simulink model "LOPES_3D"  (R2015b)
settings: Solver=ode3  StartTime=0.0  StopTime=inf  FixedStep=ts  RelTol=1e-3
PostLoadFcn:
  | DataFileTemplate = 'd:\%d_LNMC_S01_SLRT_%i.mat';
InitFcn:
  | cd(fileparts(which(gcs)));
  | runScripts
StartFcn:
  | cd(fileparts(which(gcs)));
StopFcn:
  | SaveSLRTData(DataFileTemplate)
values from neighbouring files (symbols this model uses):
  SelectorLOPESInSize = 8    [setAnkleDepInd.m]
libraries: nmc x51, simulink x22, slrtlib x14, LopesDevelopmentLibrary x7, dspsigops x1
(part 2 of 2)

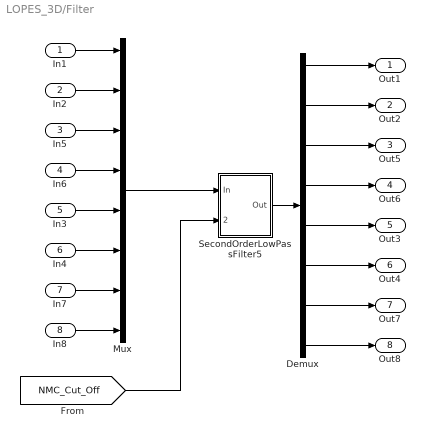
== system LOPES_3D/Filter ==
  In1 : Inport
  In2 : Inport  Port=2
  In5 : Inport  Port=3
  In6 : Inport  Port=4
  In3 : Inport  Port=5
  In4 : Inport  Port=6
  In7 : Inport  Port=7
  In8 : Inport  Port=8
  Demux : Demux  Outputs=8
  Mux : Mux  Inputs=8
  SecondOrderLowPassFilter5 : Subsystem  mask{z=0.7}
      mask prompts: z "Zeta"
  Out1 : Outport
  Out2 : Outport  Port=2
  Out5 : Outport  Port=3
  Out6 : Outport  Port=4
  Out3 : Outport  Port=5
  Out4 : Outport  Port=6
  Out7 : Outport  Port=7
  Out8 : Outport  Port=8
  wires:
  In5/1 -> Mux/3
  In2/1 -> Mux/2
  In1/1 -> Mux/1
  In6/1 -> Mux/4
  In4/1 -> Mux/6
  In3/1 -> Mux/5
  In8/1 -> Mux/8
  In7/1 -> Mux/7
  Mux/1 -> SecondOrderLowPassFilter5/1(In)
  SecondOrderLowPassFilter5/1(Out) -> Demux/1
  Demux/8 -> Out8/1
  Demux/7 -> Out7/1
  Demux/6 -> Out4/1
  Demux/5 -> Out3/1
  Demux/1 -> Out1/1
  Demux/2 -> Out2/1
  Demux/3 -> Out5/1
  Demux/4 -> Out6/1
  [NMC_Cut_Off] -> SecondOrderLowPassFilter5/2(Cut-off (hz))

== system LOPES_3D/FilterEMG ==
  In1 : Inport
  Abs1 : Abs
  SecondOrderHighPassFilter1 : Subsystem  mask{w=10*(2*pi), z=0.7}
      mask prompts: w "Cut off omega [rad/s]"; z "Zeta"
  SecondOrderLowPassFilter2 : LopesDevelopmentLibrary/Various/SecondOrderLowPassFilter  w=10*(2*pi)  z=0.7
  Out1 : Outport
  wires:
  SecondOrderLowPassFilter2/1 -> Out1/1
  Abs1/1 -> SecondOrderLowPassFilter2/1
  SecondOrderHighPassFilter1/1(Out) -> Abs1/1
  In1/1 -> SecondOrderHighPassFilter1/1(In)

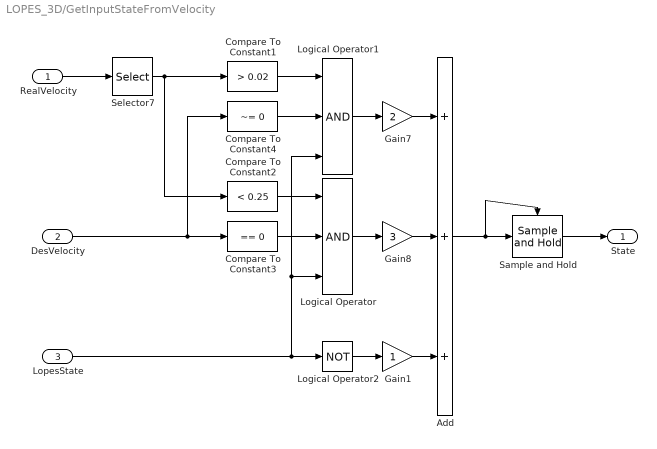
== system LOPES_3D/GetInputStateFromVelocity ==
  RealVelocity : Inport
  DesVelocity : Inport  Port=2
  LopesState : Inport  Port=3
  Add : Sum  Inputs=+++
  Compare To Constant1 : simulink/Logic and Bit Operations/Compare To Constant  relop=>  const=0.02  OutDataTypeStr=boolean
  Compare To Constant2 : simulink/Logic and Bit Operations/Compare To Constant  relop=<  const=0.25  OutDataTypeStr=boolean
  Compare To Constant3 : simulink/Logic and Bit Operations/Compare To Constant  relop===  const=0  OutDataTypeStr=boolean
  Compare To Constant4 : simulink/Logic and Bit Operations/Compare To Constant  relop=~=  const=0  OutDataTypeStr=boolean
  Gain1 : Gain  OutDataTypeStr=double
  Gain7 : Gain  Gain=2  OutDataTypeStr=double
  Gain8 : Gain  Gain=3  OutDataTypeStr=double
  Logical Operator : Logic  Inputs=3  AllPortsSameDT=off  OutDataTypeStr=boolean
  Logical Operator1 : Logic  Inputs=3  AllPortsSameDT=off  OutDataTypeStr=boolean
  Logical Operator2 : Logic  Operator=NOT  AllPortsSameDT=off  OutDataTypeStr=boolean
  Sample and Hold : dspsigops/Sample and Hold  trig=Rising edge  initCond=1  latchinput=off
  Selector7 : Selector  InputPortWidth=7  IndexOptions=Index vector (dialog)  Indices=[2]  OutputSizes=1
  State : Outport
  wires:
  RealVelocity/1 -> Selector7/1
  Selector7/1 -> Compare To Constant2/1, Compare To Constant1/1
  Compare To Constant1/1 -> Logical Operator1/1
  DesVelocity/1 -> Compare To Constant4/1, Compare To Constant3/1
  Compare To Constant3/1 -> Logical Operator/2
  Compare To Constant2/1 -> Logical Operator/1
  Compare To Constant4/1 -> Logical Operator1/2
  Logical Operator1/1 -> Gain7/1
  Logical Operator/1 -> Gain8/1
  Gain7/1 -> Add/1
  Gain8/1 -> Add/2
  Add/1 -> Sample and Hold/Trigger, Sample and Hold/1
  Sample and Hold/1 -> State/1
  LopesState/1 -> Logical Operator1/3, Logical Operator/3, Logical Operator2/1
  Gain1/1 -> Add/3
  Logical Operator2/1 -> Gain1/1

== system LOPES_3D/Label1 ==
  In1 : Inport
  Demux : Demux  Outputs=3
  EstPhase : Concatenate  NumInputs=1
  MeasPhase : Concatenate  NumInputs=1
  Mux : Mux  Inputs=3
  Speed : Concatenate  NumInputs=1
  Out1 : Outport
  wires:
  Mux/1 -> Out1/1
  In1/1 -> Demux/1
  Speed/1 -> Mux/1  "Speed"
  EstPhase/1 -> Mux/3  "EstPhase"
  MeasPhase/1 -> Mux/2  "MeasPhase"
  Demux/1 -> Speed/1
  Demux/2 -> MeasPhase/1
  Demux/3 -> EstPhase/1

== system LOPES_3D/Label4 ==
  In1 : Inport
  Demux : Demux  Outputs=2
  Mux : Mux  Inputs=2
  NMCGain : Concatenate  NumInputs=1
  PosGain : Concatenate  NumInputs=1
  Out1 : Outport
  wires:
  Mux/1 -> Out1/1
  In1/1 -> Demux/1
  PosGain/1 -> Mux/1  "PosGain"
  NMCGain/1 -> Mux/2  "NMCGain"
  Demux/1 -> PosGain/1
  Demux/2 -> NMCGain/1

== system LOPES_3D/Label5 ==
  In1 : Inport
  Angle : Concatenate  NumInputs=1
  Demux : Demux  Outputs=2
  Mux : Mux  Inputs=2
  Phase : Concatenate  NumInputs=1
  Out1 : Outport
  wires:
  Demux/2 -> Phase/1
  Demux/1 -> Angle/1
  Phase/1 -> Mux/2  "Phase"
  Angle/1 -> Mux/1  "Angle"
  In1/1 -> Demux/1
  Mux/1 -> Out1/1

== system LOPES_3D/Label6 ==
  In1 : Inport
  Demux : Demux  Outputs=2
  Force : Concatenate  NumInputs=1
  Mux : Mux  Inputs=2
  Phase : Concatenate  NumInputs=1
  Out1 : Outport
  wires:
  Mux/1 -> Out1/1
  In1/1 -> Demux/1
  Force/1 -> Mux/1  "Force"
  Phase/1 -> Mux/2  "Phase"
  Demux/1 -> Force/1
  Demux/2 -> Phase/1

== system LOPES_3D/LabelAngles ==
  In1 : Inport
  GeyerAngle : Concatenate  NumInputs=1
  Out1 : Outport
  wires:
  In1/1 -> GeyerAngle/1
  GeyerAngle/1 -> Out1/1  "GeyerAngle"

== system LOPES_3D/LabelEMG ==
  Sigs : Inport
  Demux : Demux  Outputs=8
  M{1..8} (8 alike) : Concatenate  NumInputs=1
  Mux1 : Mux  Inputs=8
  LabSigs : Outport
  wires:
  Sigs/1 -> Demux/1
  Demux/1 -> M1/1
  Demux/2 -> M2/1
  Mux1/1 -> LabSigs/1
  Demux/3 -> M3/1
  Demux/4 -> M4/1
  Demux/5 -> M5/1
  Demux/6 -> M6/1
  Demux/7 -> M7/1
  Demux/8 -> M8/1
  M2/1 -> Mux1/2  "M2"
  M1/1 -> Mux1/1  "M1"
  M6/1 -> Mux1/6  "M6"
  M7/1 -> Mux1/7  "M7"
  M3/1 -> Mux1/3  "M3"
  M5/1 -> Mux1/5  "M5"
  M4/1 -> Mux1/4  "M4"
  M8/1 -> Mux1/8  "M8"

== system LOPES_3D/LabelPhase ==
  Sigs : Inport
  Demux : Demux  Outputs=3
  EstPhase : Concatenate  NumInputs=1
  MeasPhase : Concatenate  NumInputs=1
  Mux : Mux  Inputs=3
  Speed : Concatenate  NumInputs=1
  LabSigs : Outport
  wires:
  Demux/3 -> EstPhase/1
  Demux/2 -> MeasPhase/1
  Demux/1 -> Speed/1
  MeasPhase/1 -> Mux/2  "MeasPhase"
  EstPhase/1 -> Mux/3  "EstPhase"
  Speed/1 -> Mux/1  "Speed"
  Sigs/1 -> Demux/1
  Mux/1 -> LabSigs/1

== system LOPES_3D/LabelTorque ==
  In1 : Inport
  NMCTorquePure : Concatenate  NumInputs=1
  Out1 : Outport
  wires:
  NMCTorquePure/1 -> Out1/1  "NMCTorquePure"
  In1/1 -> NMCTorquePure/1

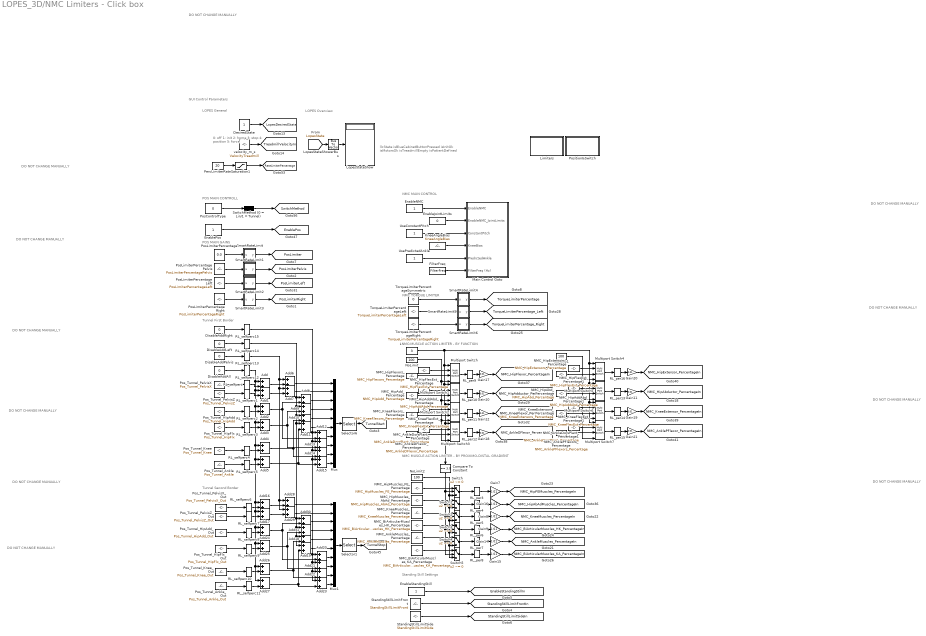
== system LOPES_3D/NMC Limiters - Click box ==
  note: Standing Still Settings
  note: GUI Control Parameters
  note: LOPES Overview
  note: llcState
      | isBlueCabinetButtonPressed
      | isInitOk
      | isMotorsOk
      | isTreadmillEmpty
      | isPatientDefined
  note: 0: off
      | 1: init
      | 2: home
      | 3: stop
      | 4: position
      | 5: force
  note: LOPES General
  note: Tunnel Second Border
  note: POS MAIN CONTROLL
  note: POS MAIN GAINS
  note: NMC MAIN CONTROL
  note: NMC TORQUE LIMITER
  note: NMC MUSCLE ACTION LIMITER - BY PROXIMO-DISTAL GRADIENT
  note: NMC MUSCLE ACTION LIMITER - BY FUNCTION
  note: Tunnel First Border
  note: DO NOT CHANGE MANUALLY
  note: DO NOT CHANGE MANUALLY
  note: DO NOT CHANGE MANUALLY
  note: DO NOT CHANGE MANUALLY
  note: DO NOT CHANGE MANUALLY
  note: DO NOT CHANGE MANUALLY
  note: DO NOT CHANGE MANUALLY
  note: DO NOT CHANGE MANUALLY
  note: DO NOT CHANGE MANUALLY
  note: DO NOT CHANGE MANUALLY
  note: DO NOT CHANGE MANUALLY
  Add{,1..31} (32 alike) : Sum
  Compare To Constant : simulink/Logic and Bit Operations/Compare To Constant  relop===  const=3.0  OutDataTypeStr=boolean
  DesiredState : Constant
  DisableAddAll : Constant  Value=0
  DisableAddLeft : Constant  Value=0
  DisableAddPelvis : Constant  Value=0
  DisableAddRight : Constant  Value=0
  EnableJointLimits : Constant  Value=0  OutDataTypeStr=double
      settings: OpenFcn=|
      | b = get_param(gcb,'value');
      | if (strcmp(b,'1')),
      |   set_param (gcb,'value','0');
      | else
      |   set_param(gcb,'value','1');
      | end;
  EnableNMC : Constant  OutDataTypeStr=double
      settings: OpenFcn=|
      | b = get_param(gcb,'value');
      | if (strcmp(b,'1')),
      |   set_param (gcb,'value','0');
      | else
      |   set_param(gcb,'value','1');
      | end;
  EnablePos : Constant  OutDataTypeStr=double
      settings: OpenFcn=|
      | b = get_param(gcb,'value');
      | if (strcmp(b,'1')),
      |   set_param (gcb,'value','0');
      | else
      |   set_param(gcb,'value','1');
      | end;
  EnableStandingStill : Constant  OutDataTypeStr=double
      settings: OpenFcn=|
      | b = get_param(gcb,'value');
      | if (strcmp(b,'1')),
      |   set_param (gcb,'value','0');
      | else
      |   set_param(gcb,'value','1');
      | end;
  FilterFreq : Constant  Value=FilterFreq
  Gain{7..12,14..21} (14 alike) : Gain  Gain=0.01
  KneeAngleBias : Constant  Value=KneeAngleBias
  LimiterMethod : Constant  Value=3
  Limiters : Subsystem
  LopesStateShow : Display
      settings: AttributesFormatString=%<Tag>
  LopesStateShowerBus : BusToVector
  Main Control Goto : Subsystem
  Multiport Switch{,1..7} (8 alike) : MultiPortSwitch
  Mux : Mux  Inputs=10
  Mux1 : Mux  Inputs=10
  NMC_AnkleDFlexor_Percentage : Constant  Value=NMC_AnkleDFlexor_Percentage
  NMC_AnkleDorsPlant_Percentage : Constant  Value=NMC_AnkleDorsPlant_Percentage
  NMC_AnkleDorsPlant_Percentage1 : Constant  Value=NMC_AnkleDorsPlant_Percentage
  NMC_AnkleMuscles_Percentage : Constant  Value=NMC_AnkleMuscles_Percentage
  NMC_AnklePFlexors_Percentage : Constant  Value=NMC_AnklePFlexors_Percentage
  NMC_BiArticularMuscles_HK_Percentage : Constant  Value=NMC_BiArticularMuscles_HK_Percentage
  NMC_BiArticularMuscles_KA_Percentage : Constant  Value=NMC_BiArticularMuscles_KA_Percentage
  NMC_HipAbd_Percentage : Constant  Value=NMC_HipAbd_Percentage
  NMC_HipAddAbd_Percentage : Constant  Value=NMC_HipAddAbd_Percentage
  NMC_HipAddAbd_Percentage1 : Constant  Value=NMC_HipAddAbd_Percentage
  NMC_HipAdd_Percentage : Constant  Value=NMC_HipAdd_Percentage
  NMC_HipExtensors_Percentage : Constant  Value=NMC_HipExtensors_Percentage
  NMC_HipFlexExt_Percentage : Constant  Value=NMC_HipFlexExt_Percentage
  NMC_HipFlexExt_Percentage1 : Constant  Value=NMC_HipFlexExt_Percentage
  NMC_HipFlexors_Percentage : Constant  Value=NMC_HipFlexors_Percentage
  NMC_HipMuscles_AbAd_Percentage : Constant  Value=NMC_HipMuscles_AbAd_Percentage
  NMC_HipMuscles_FE_Percentage : Constant  Value=NMC_HipMuscles_FE_Percentage
  NMC_KneeExtensors_Percentage : Constant  Value=NMC_KneeExtensors_Percentage
  NMC_KneeFlexExt_Percentage : Constant  Value=NMC_KneeFlexExt_Percentage
  NMC_KneeFlexExt_Percentage1 : Constant  Value=NMC_KneeFlexExt_Percentage
  NMC_KneeFlexors_Percentage : Constant  Value=NMC_KneeFlexors_Percentage
  NMC_KneeMuscles_Percentage : Constant  Value=NMC_KneeMuscles_Percentage
  NoLimit : Constant  Value=100
  NoLimit1 : Constant  Value=100
  NoLimit2 : Constant  Value=100
  PercLimiterRate : Constant  Value=20
  PosControlType : Constant  Value=0  OutDataTypeStr=double
      settings: OpenFcn=|
      | b = get_param(gcb,'value');
      | if (strcmp(b,'1')),
      |   set_param (gcb,'value','0');
      | else
      |   set_param(gcb,'value','1');
      | end;
  PosLimiterPercentage : Constant  Value=0.0
  PosLimiterPercentageLeft : Constant  Value=PosLimiterPercentageLeft
  PosLimiterPercentagePelvis : Constant  Value=PosLimiterPercentagePelvis
  PosLimiterPercentageRight : Constant  Value=PosLimiterPercentageRight
  Pos_Tunnel_Ankle : Constant  Value=Pos_Tunnel_Ankle
  Pos_Tunnel_Ankle_Out : Constant  Value=Pos_Tunnel_Ankle_Out
  Pos_Tunnel_HipAdd : Constant  Value=Pos_Tunnel_HipAdd
  Pos_Tunnel_HipAdd_Out : Constant  Value=Pos_Tunnel_HipAdd_Out
  Pos_Tunnel_HipFlx : Constant  Value=Pos_Tunnel_HipFlx
  Pos_Tunnel_HipFlx_Out : Constant  Value=Pos_Tunnel_HipFlx_Out
  Pos_Tunnel_Knee : Constant  Value=Pos_Tunnel_Knee
  Pos_Tunnel_Knee_Out : Constant  Value=Pos_Tunnel_Knee_Out
  Pos_Tunnel_PelvisX : Constant  Value=Pos_Tunnel_PelvisX
  Pos_Tunnel_PelvisX_Out : Constant  Value=Pos_Tunnel_PelvisX_Out
  Pos_Tunnel_PelvisZ : Constant  Value=Pos_Tunnel_PelvisZ
  Pos_Tunnel_PelvisZ_Out : Constant  Value=Pos_Tunnel_PelvisZ_Out
  Position&Switch : Subsystem
  RL_per{3..16} (14 alike) : nmc/RL_per
  RL_selfperc{,1..15} (16 alike) : nmc/RL_selfperc
  Saturation1 : Saturate  UpperLimit=100  LowerLimit=0
  Selector1 : Selector  InputPortWidth=10  IndexOptions=Index vector (dialog)  Indices=SelectorLOPESIn  OutputSizes=1
  Selector6 : Selector  InputPortWidth=10  IndexOptions=Index vector (dialog)  Indices=SelectorLOPESIn  OutputSizes=1
  SmartRateLimit : Subsystem
  SmartRateLimit1 : Subsystem
  SmartRateLimit2 : Subsystem
  SmartRateLimit3 : Subsystem
  SmartRateLimit4 : Subsystem
  SmartRateLimit5 : Subsystem
  SmartRateLimit6 : Subsystem
  StandingStillLimitFront : Constant  Value=StandingStillLimitFront
  StandingStillLimitSide : Constant  Value=StandingStillLimitSide
  Switch{,1..5} (6 alike) : Switch  Criteria=u2 ~= 0
  SwitchMethod (0 = Lin/1 = Tunnel) : Concatenate  NumInputs=1
  TorqueLimiterPercentageLeft : Constant  Value=TorqueLimiterPercentageLeft
  TorqueLimiterPercentageRight : Constant  Value=TorqueLimiterPercentageRight
  TorqueLimiterPercentageSymmetric : Constant  Value=0
  UseConstantPitch : Constant  OutDataTypeStr=double
      settings: OpenFcn=|
      | b = get_param(gcb,'value');
      | if (strcmp(b,'1')),
      |   set_param (gcb,'value','0');
      | else
      |   set_param(gcb,'value','1');
      | end;
  UsePredictedAnkle : Constant  OutDataTypeStr=double
      settings: OpenFcn=|
      | b = get_param(gcb,'value');
      | if (strcmp(b,'1')),
      |   set_param (gcb,'value','0');
      | else
      |   set_param(gcb,'value','1');
      | end;
  velocity_m_s : Constant  Value=VelocityTreadmill
  tag scope: EnablePos=global, EnableStandingStillIn=global, LopesDesiredState=global, NMC_AnkleDFlexor_PercentageIn=global, NMC_AnkleMuscles_PercentageIn=global, NMC_AnklePFlexor_PercentageIn=global, NMC_BiArticularMuscles_HK_PercentageIn=global, NMC_BiArticularMuscles_KA_PercentageIn=global, NMC_HipAbAdMuscles_PercentageIn=global, NMC_HipAbductor_PercentageIn=global, NMC_HipAdductor_PercentageIn=global, NMC_HipExtensor_PercentageIn=global, NMC_HipFEMuscles_PercentageIn=global, NMC_HipFlexor_PercentageIn=global, NMC_KneeExtensor_PercentageIn=global, NMC_KneeFlexor_PercentageIn=global, NMC_KneeMuscles_PercentageIn=global, PosLimiter=global, PosLimiterLeft=global, PosLimiterPelvis=global, PosLimiterRight=global, RateLimiterPercentage=global, StandingStillLimitFrontIn=global, StandingStillLimitSideIn=global, SwitchMethod=global, TorqueLimiterPercentage=global, TorqueLimiterPercentage_Left=global, TorqueLimiterPercentage_Right=global, TreadmillVelocityIn=global, TunnelStart=global, TunnelStop=global
  wires:
  Switch5/1 -> RL_per8/1
  Switch4/1 -> RL_per7/1
  Switch3/1 -> RL_per6/1
  Switch/1 -> RL_per3/1
  Switch1/1 -> RL_per4/1
  Switch2/1 -> RL_per5/1
  NMC_BiArticularMuscles_KA_Percentage/1 -> Switch5/1
  NMC_AnkleMuscles_Percentage/1 -> Switch4/1
  NMC_BiArticularMuscles_HK_Percentage/1 -> Switch3/1
  NMC_KneeMuscles_Percentage/1 -> Switch2/1
  NMC_HipMuscles_AbAd_Percentage/1 -> Switch1/1
  NoLimit2/1 -> Switch/3, Switch1/3, Switch2/3, Switch3/3, Switch4/3, Switch5/3
  NoLimit/1 -> Multiport Switch2/4, Multiport Switch3/4, Multiport Switch1/4, Multiport Switch/4
  NMC_HipFlexExt_Percentage1/1 -> Multiport Switch4/2
  NMC_HipAddAbd_Percentage1/1 -> Multiport Switch5/2
  NMC_KneeFlexExt_Percentage1/1 -> Multiport Switch6/2
  NMC_AnkleDorsPlant_Percentage1/1 -> Multiport Switch7/2
  NMC_HipFlexExt_Percentage/1 -> Multiport Switch/2
  NMC_KneeFlexExt_Percentage/1 -> Multiport Switch2/2
  NMC_AnkleDorsPlant_Percentage/1 -> Multiport Switch3/2
  NMC_HipAddAbd_Percentage/1 -> Multiport Switch1/2
  NoLimit1/1 -> Multiport Switch7/4, Multiport Switch6/4, Multiport Switch5/4, Multiport Switch4/4
  Multiport Switch7/1 -> RL_per15/1
  Multiport Switch6/1 -> RL_per14/1
  Multiport Switch5/1 -> RL_per13/1
  Multiport Switch4/1 -> RL_per16/1
  NMC_AnklePFlexors_Percentage/1 -> Multiport Switch7/3
  NMC_KneeExtensors_Percentage/1 -> Multiport Switch6/3
  NMC_HipAbd_Percentage/1 -> Multiport Switch5/3
  NMC_HipExtensors_Percentage/1 -> Multiport Switch4/3
  NMC_AnkleDFlexor_Percentage/1 -> Multiport Switch3/3
  Multiport Switch3/1 -> RL_per12/1
  Multiport Switch2/1 -> RL_per11/1
  Multiport Switch1/1 -> RL_per10/1
  Multiport Switch/1 -> RL_per9/1
  LimiterMethod/1 -> Multiport Switch4/1, Multiport Switch5/1, Multiport Switch6/1, Multiport Switch7/1, Multiport Switch2/1, Compare To Constant/1, Multiport Switch3/1, Multiport Switch1/1, Multiport Switch/1
  SmartRateLimit4/1(y) -> [TorqueLimiterPercentage]
  TorqueLimiterPercentageSymmetric/1 -> SmartRateLimit4/1(u)
  SmartRateLimit/1(y) -> [PosLimiter]
  PosLimiterPercentage/1 -> SmartRateLimit/1(u)
  StandingStillLimitFront/1 -> [StandingStillLimitFrontIn]
  StandingStillLimitSide/1 -> [StandingStillLimitSideIn]
  EnableStandingStill/1 -> [EnableStandingStillIn]
  [LopesState] -> LopesStateShowerBus/1
  LopesStateShowerBus/1 -> LopesStateShow/1
  DesiredState/1 -> [LopesDesiredState]
  velocity_m_s/1 -> [TreadmillVelocityIn]
  Mux1/1 -> Selector1/1
  Pos_Tunnel_PelvisX_Out/1 -> RL_selfperc6/1
  Pos_Tunnel_Ankle_Out/1 -> RL_selfperc11/1
  Pos_Tunnel_Knee_Out/1 -> RL_selfperc10/1
  Pos_Tunnel_HipFlx_Out/1 -> RL_selfperc9/1
  Pos_Tunnel_HipAdd_Out/1 -> RL_selfperc8/1
  Pos_Tunnel_PelvisZ_Out/1 -> RL_selfperc7/1
  RL_selfperc/1 -> Add/2
  RL_selfperc1/1 -> Add1/2
  Mux/1 -> Selector6/1
  Pos_Tunnel_PelvisX/1 -> RL_selfperc/1
  Selector6/1 -> [TunnelStart]
  Pos_Tunnel_Ankle/1 -> RL_selfperc5/1
  Pos_Tunnel_Knee/1 -> RL_selfperc4/1
  Pos_Tunnel_HipFlx/1 -> RL_selfperc3/1
  Pos_Tunnel_HipAdd/1 -> RL_selfperc2/1
  Pos_Tunnel_PelvisZ/1 -> RL_selfperc1/1
  EnablePos/1 -> [EnablePos]
  SwitchMethod (0 = Lin/1 = Tunnel)/1 -> [SwitchMethod]
  Saturation1/1 -> [RateLimiterPercentage]
  PercLimiterRate/1 -> Saturation1/1
  Selector1/1 -> [TunnelStop]
  PosControlType/1 -> SwitchMethod (0 = Lin/1 = Tunnel)/1
  SmartRateLimit1/1(y) -> [PosLimiterPelvis]
  PosLimiterPercentagePelvis/1 -> SmartRateLimit1/1(u)
  PosLimiterPercentageRight/1 -> SmartRateLimit3/1(u)
  SmartRateLimit3/1(y) -> [PosLimiterRight]
  SmartRateLimit2/1(y) -> [PosLimiterLeft]
  PosLimiterPercentageLeft/1 -> SmartRateLimit2/1(u)
  FilterFreq/1 -> Main Control Goto/6(FilterFreq (Hz))
  UsePredictedAnkle/1 -> Main Control Goto/5(PredictedAnkle)
  KneeAngleBias/1 -> Main Control Goto/4("KneeBias ")
  UseConstantPitch/1 -> Main Control Goto/3(ConstantPitch)
  EnableJointLimits/1 -> Main Control Goto/2(EnableNMC_JointLimits)
  EnableNMC/1 -> Main Control Goto/1(EnableNMC)
  TorqueLimiterPercentageRight/1 -> SmartRateLimit6/1(u)
  TorqueLimiterPercentageLeft/1 -> SmartRateLimit5/1(u)
  RL_per8/1 -> Gain15/1
  RL_per7/1 -> Gain14/1
  RL_per6/1 -> Gain9/1
  RL_per5/1 -> Gain8/1
  RL_per4/1 -> Gain16/1
  RL_per3/1 -> Gain7/1
  Gain16/1 -> [NMC_HipAbAdMuscles_PercentageIn]
  Gain15/1 -> [NMC_BiArticularMuscles_KA_PercentageIn]
  Gain14/1 -> [NMC_AnkleMuscles_PercentageIn]
  Gain9/1 -> [NMC_BiArticularMuscles_HK_PercentageIn]
  Gain8/1 -> [NMC_KneeMuscles_PercentageIn]
  Gain7/1 -> [NMC_HipFEMuscles_PercentageIn]
  NMC_HipMuscles_FE_Percentage/1 -> Switch/1
  RL_per15/1 -> Gain21/1
  RL_per14/1 -> Gain19/1
  RL_per16/1 -> Gain20/1
  RL_per13/1 -> Gain11/1
  RL_per12/1 -> Gain18/1
  RL_per11/1 -> Gain12/1
  NMC_KneeFlexors_Percentage/1 -> Multiport Switch2/3
  RL_per10/1 -> Gain10/1
  NMC_HipAdd_Percentage/1 -> Multiport Switch1/3
  RL_per9/1 -> Gain17/1
  NMC_HipFlexors_Percentage/1 -> Multiport Switch/3
  Gain11/1 -> [NMC_HipAbductor_PercentageIn]
  Gain10/1 -> [NMC_HipAdductor_PercentageIn]
  Gain21/1 -> [NMC_AnklePFlexor_PercentageIn]
  Gain20/1 -> [NMC_HipExtensor_PercentageIn]
  Gain19/1 -> [NMC_KneeExtensor_PercentageIn]
  Gain18/1 -> [NMC_AnkleDFlexor_PercentageIn]
  Gain17/1 -> [NMC_HipFlexor_PercentageIn]
  Gain12/1 -> [NMC_KneeFlexor_PercentageIn]
  Compare To Constant/1 -> Switch5/2, Switch4/2, Switch3/2, Switch2/2, Switch1/2, Switch/2
  DisableAddAll/1 -> RL_selfperc12/1
  DisableAddPelvis/1 -> RL_selfperc13/1
  DisableAddLeft/1 -> RL_selfperc14/1
  DisableAddRight/1 -> RL_selfperc15/1
  Add/1 -> Add6/2
  RL_selfperc2/1 -> Add2/2
  Add2/1 -> Add12/2, Add8/2
  RL_selfperc3/1 -> Add3/2
  Add3/1 -> Add9/2, Add13/2
  RL_selfperc4/1 -> Add4/2
  Add4/1 -> Add14/2, Add10/2
  RL_selfperc5/1 -> Add5/2
  Add5/1 -> Add15/2, Add11/2
  Add6/1 -> Mux/1
  Add1/1 -> Add7/2
  Add7/1 -> Mux/2
  Add8/1 -> Mux/3
  Add9/1 -> Mux/4
  Add10/1 -> Mux/5
  Add11/1 -> Mux/6
  Add12/1 -> Mux/7
  Add13/1 -> Mux/8
  Add14/1 -> Mux/9
  Add15/1 -> Mux/10
  RL_selfperc6/1 -> Add16/2
  RL_selfperc7/1 -> Add17/2
  Add16/1 -> Add28/2
  RL_selfperc12/1 -> Add1/1, Add16/1, Add24/1, Add25/1, Add26/1, Add27/1, Add17/1, Add5/1, Add4/1, Add3/1, Add2/1, Add/1
  RL_selfperc8/1 -> Add24/2
  Add24/1 -> Add30/2, Add20/2
  RL_selfperc9/1 -> Add25/2
  Add25/1 -> Add21/2, Add31/2
  RL_selfperc10/1 -> Add26/2
  Add26/1 -> Add18/2, Add22/2
  RL_selfperc11/1 -> Add27/2
  Add27/1 -> Add19/2, Add23/2
  RL_selfperc13/1 -> Add28/1, Add29/1, Add7/1, Add6/1
  Add28/1 -> Mux1/1
  Add17/1 -> Add29/2
  Add29/1 -> Mux1/2
  RL_selfperc14/1 -> Add30/1, Add31/1, Add18/1, Add19/1, Add11/1, Add10/1, Add9/1, Add8/1
  Add30/1 -> Mux1/3
  Add31/1 -> Mux1/4
  Add18/1 -> Mux1/5
  Add19/1 -> Mux1/6
  Add20/1 -> Mux1/7
  Add21/1 -> Mux1/8
  Add22/1 -> Mux1/9
  Add23/1 -> Mux1/10
  RL_selfperc15/1 -> Add20/1, Add21/1, Add22/1, Add23/1, Add15/1, Add14/1, Add13/1, Add12/1
  SmartRateLimit5/1(y) -> [TorqueLimiterPercentage_Left]
  SmartRateLimit6/1(y) -> [TorqueLimiterPercentage_Right]

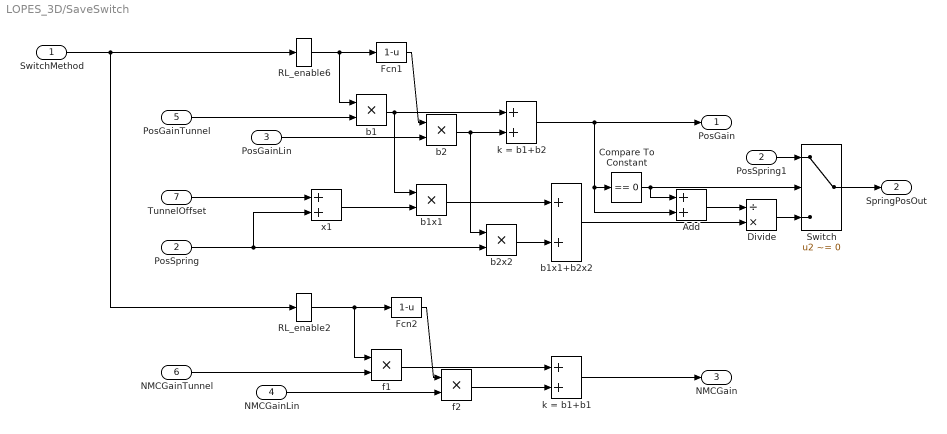
== system LOPES_3D/SaveSwitch ==
  SwitchMethod : Inport
  PosSpring : Inport  Port=2
  PosGainLin : Inport  Port=3
  NMCGainLin : Inport  Port=4
  PosGainTunnel : Inport  Port=5
  NMCGainTunnel : Inport  Port=6
  "TunnelOffset " : Inport  Port=7
  Add : Sum
  Compare To Constant : simulink/Logic and Bit Operations/Compare To Constant  relop===  const=0  OutDataTypeStr=boolean
  Divide : Product  Inputs=/*
  Fcn1 : Fcn  Expr=1-u
  Fcn2 : Fcn  Expr=1-u
  PosSpring1 : InportShadow  Port=2
  RL_enable2 : nmc/RL_enable
  RL_enable6 : nmc/RL_enable
  Switch : Switch  Criteria=u2 ~= 0
  b1 : Product
  b1x1 : Product
  b1x1+b2x2 : Sum
  b2 : Product
  b2x2 : Product
  f1 : Product
  f2 : Product
  k = b1+b1 : Sum
  k = b1+b2 : Sum
  x1 : Sum
  PosGain : Outport
  SpringPosOut : Outport  Port=2
  NMCGain : Outport  Port=3
  wires:
  RL_enable6/1 -> b1/1, Fcn1/1
  k = b1+b2/1 -> PosGain/1, Add/2, Compare To Constant/1
  NMCGainTunnel/1 -> f1/2
  b1x1+b2x2/1 -> Divide/2
  f1/1 -> k = b1+b1/1
  b2x2/1 -> b1x1+b2x2/2
  "TunnelOffset "/1 -> x1/1
  PosSpring/1 -> x1/2, b2x2/2
  x1/1 -> b1x1/2
  SwitchMethod/1 -> RL_enable2/1, RL_enable6/1
  Fcn2/1 -> f2/1
  RL_enable2/1 -> Fcn2/1, f1/1
  NMCGainLin/1 -> f2/2
  b2/1 -> b2x2/1, k = b1+b2/2
  b1x1/1 -> b1x1+b2x2/1
  b1/1 -> b1x1/1, k = b1+b2/1
  k = b1+b1/1 -> NMCGain/1
  f2/1 -> k = b1+b1/2
  PosGainTunnel/1 -> b1/2
  Fcn1/1 -> b2/1
  PosGainLin/1 -> b2/2
  Compare To Constant/1 -> Switch/2, Add/1
  Switch/1 -> SpringPosOut/1
  PosSpring1/1 -> Switch/1
  Divide/1 -> Switch/3
  Add/1 -> Divide/1

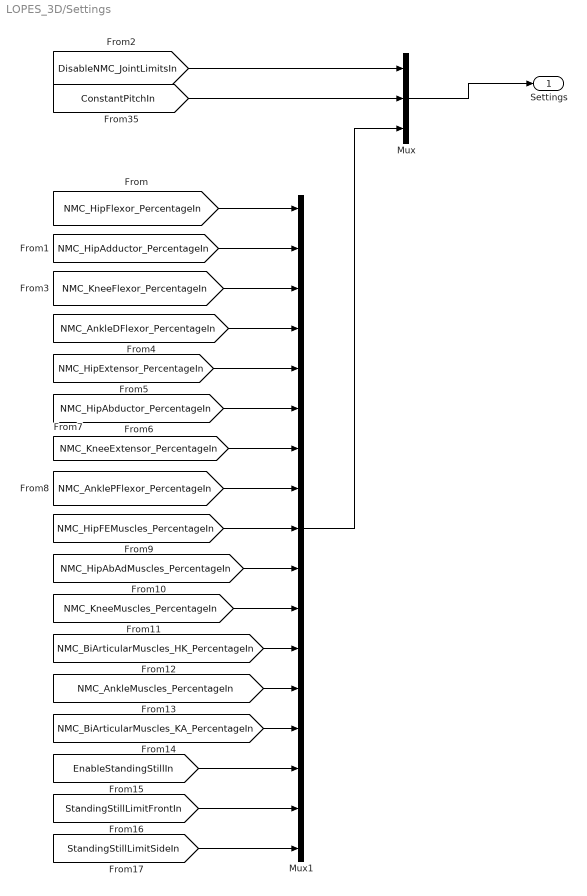
== system LOPES_3D/Settings ==
  Mux : Mux  Inputs=3
  Mux1 : Mux  Inputs=17
  Settings : Outport
  wires:
  [ConstantPitchIn] -> Mux/2
  [DisableNMC_JointLimitsIn] -> Mux/1
  Mux/1 -> Settings/1
  [NMC_BiArticularMuscles_HK_PercentageIn] -> Mux1/12
  [NMC_BiArticularMuscles_KA_PercentageIn] -> Mux1/14
  [NMC_AnkleMuscles_PercentageIn] -> Mux1/13
  [NMC_HipAbAdMuscles_PercentageIn] -> Mux1/10
  [NMC_HipAdductor_PercentageIn] -> Mux1/2
  [NMC_HipFEMuscles_PercentageIn] -> Mux1/9
  [NMC_AnklePFlexor_PercentageIn] -> Mux1/8
  [NMC_KneeFlexor_PercentageIn] -> Mux1/3
  [NMC_AnkleDFlexor_PercentageIn] -> Mux1/4
  [NMC_HipAbductor_PercentageIn] -> Mux1/6
  [NMC_KneeMuscles_PercentageIn] -> Mux1/11
  [NMC_HipExtensor_PercentageIn] -> Mux1/5
  [NMC_KneeExtensor_PercentageIn] -> Mux1/7
  [NMC_HipFlexor_PercentageIn] -> Mux1/1
  Mux1/1 -> Mux/3
  [EnableStandingStillIn] -> Mux1/15
  [StandingStillLimitFrontIn] -> Mux1/16
  [StandingStillLimitSideIn] -> Mux1/17

== system LOPES_3D/Simple Linear Switch ==
  ones : Constant  Value=ones(SelectorLOPESInSize,1)
  pos_gain : Outport
  NMC_gain : Outport  Port=2
  wires:
  ones/1 -> NMC_gain/1, pos_gain/1

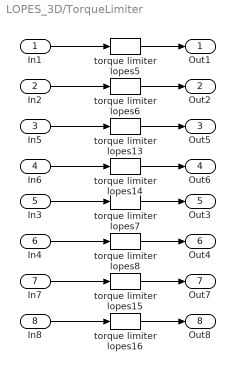
== system LOPES_3D/TorqueLimiter ==
  In1 : Inport
  In2 : Inport  Port=2
  In5 : Inport  Port=3
  In6 : Inport  Port=4
  In3 : Inport  Port=5
  In4 : Inport  Port=6
  In7 : Inport  Port=7
  In8 : Inport  Port=8
  torque limiter lopes{5..6,13..14} (4 alike) : nmc/torque limiter lopes  TorqueLimiterPercentage=TorqueLimiterPercentage_Right
  torque limiter lopes{7..8,15..16} (4 alike) : nmc/torque limiter lopes  TorqueLimiterPercentage=TorqueLimiterPercentage_Left
  Out1 : Outport
  Out2 : Outport  Port=2
  Out5 : Outport  Port=3
  Out6 : Outport  Port=4
  Out3 : Outport  Port=5
  Out4 : Outport  Port=6
  Out7 : Outport  Port=7
  Out8 : Outport  Port=8
  wires:
  In1/1 -> torque limiter lopes5/1
  In3/1 -> torque limiter lopes7/1
  In2/1 -> torque limiter lopes6/1
  In4/1 -> torque limiter lopes8/1
  torque limiter lopes5/1 -> Out1/1
  torque limiter lopes6/1 -> Out2/1
  torque limiter lopes7/1 -> Out3/1
  torque limiter lopes8/1 -> Out4/1
  In5/1 -> torque limiter lopes13/1
  In7/1 -> torque limiter lopes15/1
  In6/1 -> torque limiter lopes14/1
  In8/1 -> torque limiter lopes16/1
  torque limiter lopes13/1 -> Out5/1
  torque limiter lopes14/1 -> Out6/1
  torque limiter lopes15/1 -> Out7/1
  torque limiter lopes16/1 -> Out8/1

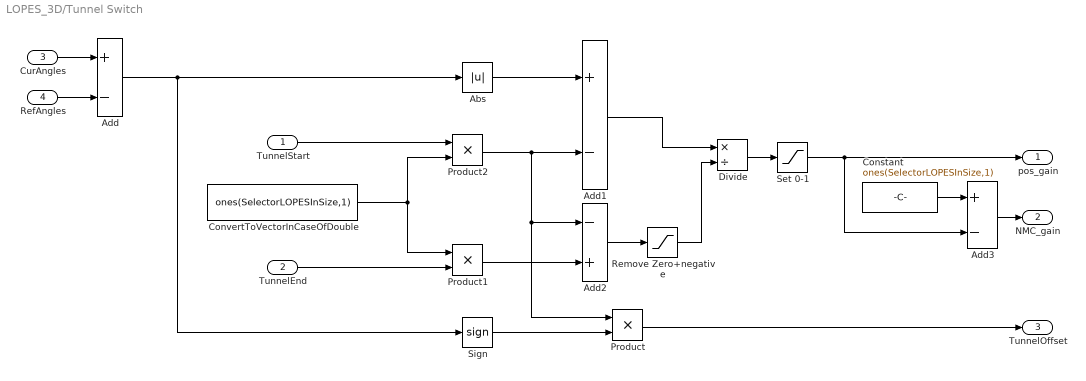
== system LOPES_3D/Tunnel Switch ==
  TunnelStart : Inport
  TunnelEnd : Inport  Port=2
  CurAngles : Inport  Port=3
  RefAngles : Inport  Port=4
  Abs : Abs
  Add : Sum  Inputs=+-
  Add1 : Sum  Inputs=+-
  Add2 : Sum  Inputs=-+
  Add3 : Sum  Inputs=+-
  Constant : Constant  Value=ones(SelectorLOPESInSize,1)
  ConvertToVectorInCaseOfDouble : Constant  Value=ones(SelectorLOPESInSize,1)
  Divide : Product  Inputs=*/
  Product : Product
  Product1 : Product
  Product2 : Product
  Remove Zero+negative : Saturate  UpperLimit=inf  LowerLimit=0.00001  LinearizeAsGain=off
  "Set 0-1 " : Saturate  UpperLimit=1  LowerLimit=0  LinearizeAsGain=off
  Sign : Signum
  pos_gain : Outport
  NMC_gain : Outport  Port=2
  TunnelOffset : Outport  Port=3
  wires:
  CurAngles/1 -> Add/1
  RefAngles/1 -> Add/2
  Add/1 -> Abs/1, Sign/1
  Abs/1 -> Add1/1
  Add1/1 -> Divide/1
  Divide/1 -> "Set 0-1 "/1
  "Set 0-1 "/1 -> pos_gain/1, Add3/2
  Add2/1 -> Remove Zero+negative/1
  Remove Zero+negative/1 -> Divide/2
  Constant/1 -> Add3/1
  Add3/1 -> NMC_gain/1
  Sign/1 -> Product/2
  Product/1 -> TunnelOffset/1
  TunnelEnd/1 -> Product1/2
  ConvertToVectorInCaseOfDouble/1 -> Product1/1, Product2/2
  Product1/1 -> Add2/2
  TunnelStart/1 -> Product2/1
  Product2/1 -> Product/1, Add2/1, Add1/2

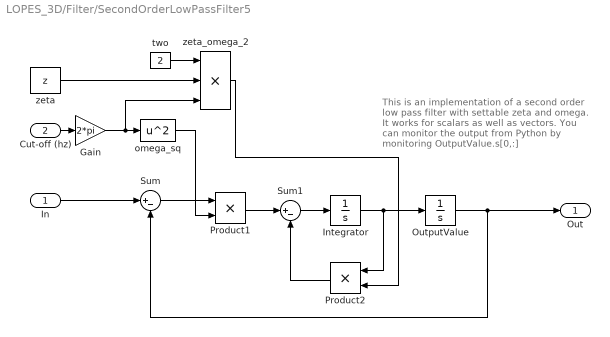
== system LOPES_3D/Filter/SecondOrderLowPassFilter5 ==
  note: This is an implementation of a
      | second order low pass filter with
      | settable zeta and omega.
      | It works for scalars as well as vectors.
      |
      | You can monitor the output from Python
      | by monitoring OutputValue.s[0,:]
  In : Inport
  Cut-off (hz) : Inport  Port=2
  Gain : Gain  Gain=2*pi
  Integrator : Integrator
  OutputValue : Integrator
  Product1 : Product  RndMeth=Zero
  Product2 : Product  RndMeth=Zero
  Sum : Sum  Inputs=|+-
  Sum1 : Sum  Inputs=|+-
  omega_sq : Math  Operator=square  SaturateOnIntegerOverflow=on
  two : Constant  Value=2
  zeta : Constant  Value=z
  zeta_omega_2 : Product  Inputs=3  RndMeth=Zero
  Out : Outport
  wires:
  Product2/1 -> Sum1/2
  zeta_omega_2/1 -> Product2/2
  Product1/1 -> Sum1/1
  omega_sq/1 -> Product1/2
  zeta/1 -> zeta_omega_2/2
  two/1 -> zeta_omega_2/1
  Cut-off (hz)/1 -> Gain/1
  Sum/1 -> Product1/1
  Integrator/1 -> OutputValue/1, Product2/1
  In/1 -> Sum/1
  Sum1/1 -> Integrator/1
  OutputValue/1 -> Sum/2, Out/1
  Gain/1 -> omega_sq/1, zeta_omega_2/3

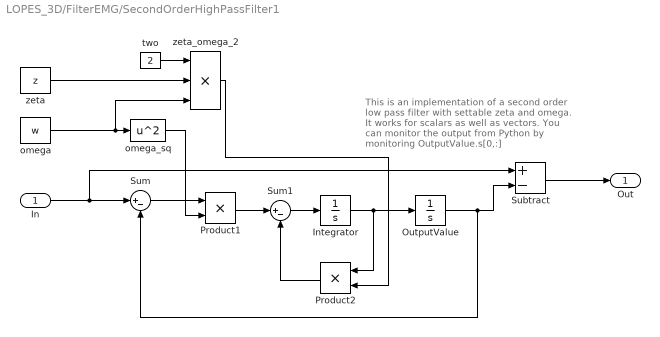
== system LOPES_3D/FilterEMG/SecondOrderHighPassFilter1 ==
  note: This is an implementation of a
      | second order low pass filter with
      | settable zeta and omega.
      | It works for scalars as well as vectors.
      |
      | You can monitor the output from Python
      | by monitoring OutputValue.s[0,:]
  In : Inport
  Integrator : Integrator
  OutputValue : Integrator
  Product1 : Product  RndMeth=Zero
  Product2 : Product  RndMeth=Zero
  Subtract : Sum  Inputs=+-
  Sum : Sum  Inputs=|+-
  Sum1 : Sum  Inputs=|+-
  omega : Constant  Value=w
  omega_sq : Math  Operator=square  SaturateOnIntegerOverflow=on
  two : Constant  Value=2
  zeta : Constant  Value=z
  zeta_omega_2 : Product  Inputs=3  RndMeth=Zero
  Out : Outport
  wires:
  Product2/1 -> Sum1/2
  zeta_omega_2/1 -> Product2/2
  Product1/1 -> Sum1/1
  omega_sq/1 -> Product1/2
  zeta/1 -> zeta_omega_2/2
  two/1 -> zeta_omega_2/1
  omega/1 -> omega_sq/1, zeta_omega_2/3
  Sum/1 -> Product1/1
  Integrator/1 -> OutputValue/1, Product2/1
  In/1 -> Subtract/1, Sum/1
  Sum1/1 -> Integrator/1
  OutputValue/1 -> Subtract/2, Sum/2
  Subtract/1 -> Out/1

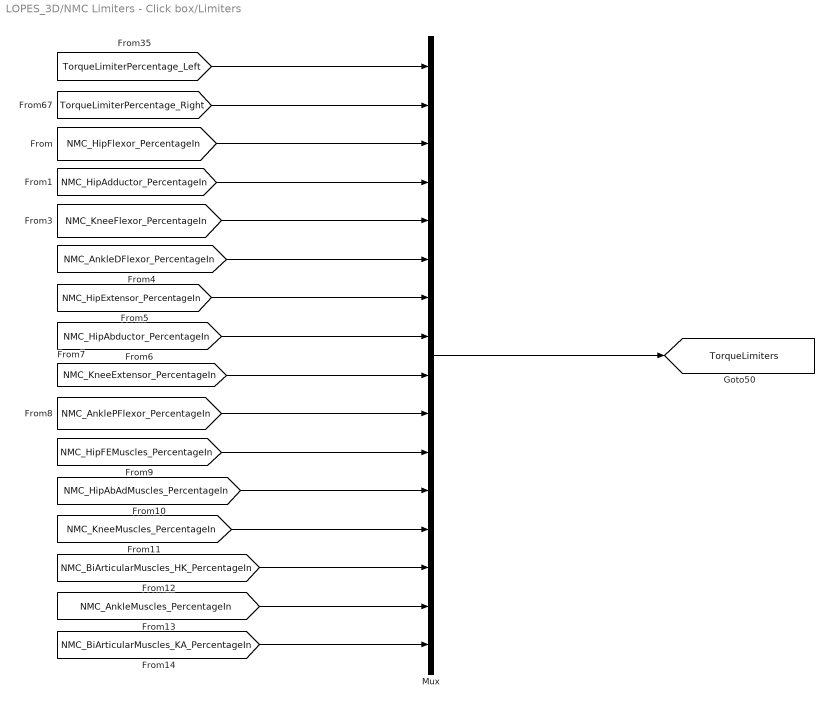
== system LOPES_3D/NMC Limiters - Click box/Limiters ==
  Mux : Mux  Inputs=16
  tag scope: TorqueLimiters=global
  wires:
  [NMC_HipExtensor_PercentageIn] -> Mux/7
  [TorqueLimiterPercentage_Left] -> Mux/1
  [NMC_HipAdductor_PercentageIn] -> Mux/4
  [NMC_HipFlexor_PercentageIn] -> Mux/3
  [TorqueLimiterPercentage_Right] -> Mux/2
  [NMC_AnklePFlexor_PercentageIn] -> Mux/10
  [NMC_KneeFlexor_PercentageIn] -> Mux/5
  [NMC_HipFEMuscles_PercentageIn] -> Mux/11
  [NMC_HipAbductor_PercentageIn] -> Mux/8
  [NMC_AnkleDFlexor_PercentageIn] -> Mux/6
  [NMC_KneeExtensor_PercentageIn] -> Mux/9
  [NMC_KneeMuscles_PercentageIn] -> Mux/13
  [NMC_HipAbAdMuscles_PercentageIn] -> Mux/12
  [NMC_AnkleMuscles_PercentageIn] -> Mux/15
  [NMC_BiArticularMuscles_HK_PercentageIn] -> Mux/14
  [NMC_BiArticularMuscles_KA_PercentageIn] -> Mux/16
  Mux/1 -> [TorqueLimiters]

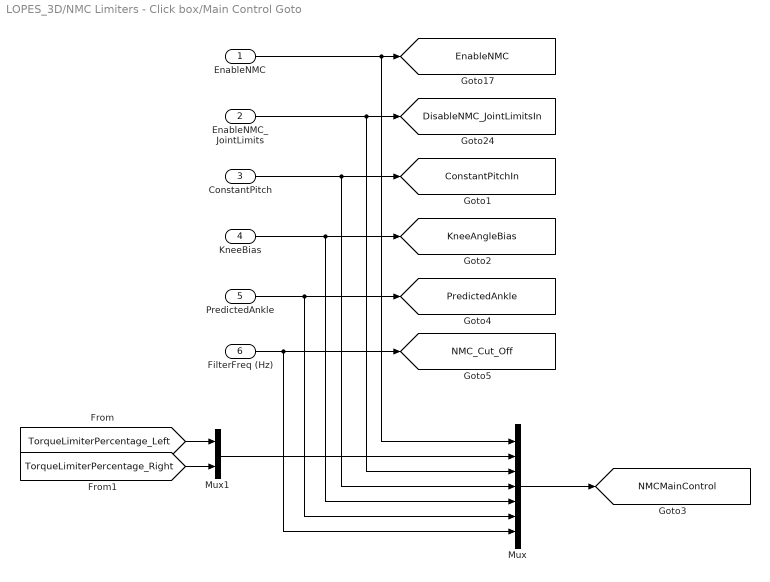
== system LOPES_3D/NMC Limiters - Click box/Main Control Goto ==
  EnableNMC : Inport
  EnableNMC_JointLimits : Inport  Port=2
  ConstantPitch : Inport  Port=3
  "KneeBias " : Inport  Port=4
  PredictedAnkle : Inport  Port=5
  FilterFreq (Hz) : Inport  Port=6
  Mux : Mux  Inputs=7
  Mux1 : Mux  Inputs=2
  tag scope: ConstantPitchIn=global, DisableNMC_JointLimitsIn=global, EnableNMC=global, KneeAngleBias=global, NMCMainControl=global, NMC_Cut_Off=global, PredictedAnkle=global
  wires:
  Mux1/1 -> Mux/2
  [TorqueLimiterPercentage_Left] -> Mux1/1
  [TorqueLimiterPercentage_Right] -> Mux1/2
  FilterFreq (Hz)/1 -> [NMC_Cut_Off], Mux/7
  PredictedAnkle/1 -> [PredictedAnkle], Mux/6
  Mux/1 -> [NMCMainControl]
  "KneeBias "/1 -> [KneeAngleBias], Mux/5
  ConstantPitch/1 -> [ConstantPitchIn], Mux/4
  EnableNMC/1 -> [EnableNMC], Mux/1
  EnableNMC_JointLimits/1 -> [DisableNMC_JointLimitsIn], Mux/3

== system LOPES_3D/NMC Limiters - Click box/Position&Switch ==
  Mux : Mux
  Mux1 : Mux  Inputs=3
  tag scope: PosSwitchSettings=global
  wires:
  Mux1/1 -> Mux/2
  [PosLimiterRight] -> Mux1/3
  [PosLimiterLeft] -> Mux1/2
  [PosLimiterPelvis] -> Mux1/1
  [NMCBiasForceGain] -> Mux/4
  [PosSpringGain] -> Mux/3
  [EnablePos] -> Mux/1
  Mux/1 -> [PosSwitchSettings]

== system LOPES_3D/NMC Limiters - Click box/SmartRateLimit ==
  u : Inport
  Compare To Constant : simulink/Logic and Bit Operations/Compare To Constant  relop=~=  const=5  OutDataTypeStr=boolean
  RateLimiterWithReset : Subsystem
  zero : Constant  Value=0
  y : Outport
  wires:
  u/1 -> RateLimiterWithReset/1(u)
  RateLimiterWithReset/1(y) -> y/1
  [RateLimiterPercentage] -> RateLimiterWithReset/2(rate)
  zero/1 -> RateLimiterWithReset/3(initial_value)
  Compare To Constant/1 -> RateLimiterWithReset/4(reset_high_active)
  [LopesLLCState] -> Compare To Constant/1

== system LOPES_3D/NMC Limiters - Click box/SmartRateLimit1 ==
  u : Inport
  Compare To Constant : simulink/Logic and Bit Operations/Compare To Constant  relop=~=  const=5  OutDataTypeStr=boolean
  RateLimiterWithReset : Subsystem
  zero : Constant  Value=0
  y : Outport
  wires:
  [LopesLLCState] -> Compare To Constant/1
  Compare To Constant/1 -> RateLimiterWithReset/4(reset_high_active)
  zero/1 -> RateLimiterWithReset/3(initial_value)
  [RateLimiterPercentage] -> RateLimiterWithReset/2(rate)
  RateLimiterWithReset/1(y) -> y/1
  u/1 -> RateLimiterWithReset/1(u)

== system LOPES_3D/NMC Limiters - Click box/SmartRateLimit2 ==
  u : Inport
  Compare To Constant : simulink/Logic and Bit Operations/Compare To Constant  relop=~=  const=5  OutDataTypeStr=boolean
  RateLimiterWithReset : Subsystem
  zero : Constant  Value=0
  y : Outport
  wires:
  u/1 -> RateLimiterWithReset/1(u)
  RateLimiterWithReset/1(y) -> y/1
  [RateLimiterPercentage] -> RateLimiterWithReset/2(rate)
  zero/1 -> RateLimiterWithReset/3(initial_value)
  Compare To Constant/1 -> RateLimiterWithReset/4(reset_high_active)
  [LopesLLCState] -> Compare To Constant/1

== system LOPES_3D/NMC Limiters - Click box/SmartRateLimit3 ==
  u : Inport
  Compare To Constant : simulink/Logic and Bit Operations/Compare To Constant  relop=~=  const=5  OutDataTypeStr=boolean
  RateLimiterWithReset : Subsystem
  zero : Constant  Value=0
  y : Outport
  wires:
  [LopesLLCState] -> Compare To Constant/1
  Compare To Constant/1 -> RateLimiterWithReset/4(reset_high_active)
  zero/1 -> RateLimiterWithReset/3(initial_value)
  [RateLimiterPercentage] -> RateLimiterWithReset/2(rate)
  RateLimiterWithReset/1(y) -> y/1
  u/1 -> RateLimiterWithReset/1(u)

== system LOPES_3D/NMC Limiters - Click box/SmartRateLimit4 ==
  u : Inport
  Compare To Constant : simulink/Logic and Bit Operations/Compare To Constant  relop=~=  const=5  OutDataTypeStr=boolean
  RateLimiterWithReset : Subsystem
  zero : Constant  Value=0
  y : Outport
  wires:
  [LopesLLCState] -> Compare To Constant/1
  Compare To Constant/1 -> RateLimiterWithReset/4(reset_high_active)
  zero/1 -> RateLimiterWithReset/3(initial_value)
  [RateLimiterPercentage] -> RateLimiterWithReset/2(rate)
  RateLimiterWithReset/1(y) -> y/1
  u/1 -> RateLimiterWithReset/1(u)

== system LOPES_3D/NMC Limiters - Click box/SmartRateLimit5 ==
  u : Inport
  Compare To Constant : simulink/Logic and Bit Operations/Compare To Constant  relop=~=  const=5  OutDataTypeStr=boolean
  RateLimiterWithReset : Subsystem
  zero : Constant  Value=0
  y : Outport
  wires:
  u/1 -> RateLimiterWithReset/1(u)
  RateLimiterWithReset/1(y) -> y/1
  [RateLimiterPercentage] -> RateLimiterWithReset/2(rate)
  zero/1 -> RateLimiterWithReset/3(initial_value)
  Compare To Constant/1 -> RateLimiterWithReset/4(reset_high_active)
  [LopesLLCState] -> Compare To Constant/1

== system LOPES_3D/NMC Limiters - Click box/SmartRateLimit6 ==
  u : Inport
  Compare To Constant : simulink/Logic and Bit Operations/Compare To Constant  relop=~=  const=5  OutDataTypeStr=boolean
  RateLimiterWithReset : Subsystem
  zero : Constant  Value=0
  y : Outport
  wires:
  [LopesLLCState] -> Compare To Constant/1
  Compare To Constant/1 -> RateLimiterWithReset/4(reset_high_active)
  zero/1 -> RateLimiterWithReset/3(initial_value)
  [RateLimiterPercentage] -> RateLimiterWithReset/2(rate)
  RateLimiterWithReset/1(y) -> y/1
  u/1 -> RateLimiterWithReset/1(u)

== system LOPES_3D/NMC Limiters - Click box/SmartRateLimit/RateLimiterWithReset ==
  u : Inport
  rate : Inport  Port=2
  initial_value : Inport  Port=3
  reset_high_active : Inport  Port=4
  Rate Limiter Dynamic : simulink/Discontinuities/Rate Limiter Dynamic
  Switch : Switch  Criteria=u2 ~= 0
  Switch1 : Switch  Criteria=u2 ~= 0
  Unary Minus : UnaryMinus
  huge : Constant  Value=1e300
  y : Outport
  wires:
  Switch/1 -> Rate Limiter Dynamic/2
  Unary Minus/1 -> Rate Limiter Dynamic/3
  Switch1/1 -> Unary Minus/1, Rate Limiter Dynamic/1
  huge/1 -> Switch1/1
  reset_high_active/1 -> Switch/2, Switch1/2
  initial_value/1 -> Switch/1
  rate/1 -> Switch1/3
  Rate Limiter Dynamic/1 -> y/1
  u/1 -> Switch/3

== system LOPES_3D/NMC Limiters - Click box/SmartRateLimit1/RateLimiterWithReset ==
  u : Inport
  rate : Inport  Port=2
  initial_value : Inport  Port=3
  reset_high_active : Inport  Port=4
  Rate Limiter Dynamic : simulink/Discontinuities/Rate Limiter Dynamic
  Switch : Switch  Criteria=u2 ~= 0
  Switch1 : Switch  Criteria=u2 ~= 0
  Unary Minus : UnaryMinus
  huge : Constant  Value=1e300
  y : Outport
  wires:
  u/1 -> Switch/3
  Rate Limiter Dynamic/1 -> y/1
  rate/1 -> Switch1/3
  initial_value/1 -> Switch/1
  reset_high_active/1 -> Switch1/2, Switch/2
  huge/1 -> Switch1/1
  Switch1/1 -> Rate Limiter Dynamic/1, Unary Minus/1
  Unary Minus/1 -> Rate Limiter Dynamic/3
  Switch/1 -> Rate Limiter Dynamic/2

== system LOPES_3D/NMC Limiters - Click box/SmartRateLimit2/RateLimiterWithReset ==
  u : Inport
  rate : Inport  Port=2
  initial_value : Inport  Port=3
  reset_high_active : Inport  Port=4
  Rate Limiter Dynamic : simulink/Discontinuities/Rate Limiter Dynamic
  Switch : Switch  Criteria=u2 ~= 0
  Switch1 : Switch  Criteria=u2 ~= 0
  Unary Minus : UnaryMinus
  huge : Constant  Value=1e300
  y : Outport
  wires:
  Switch/1 -> Rate Limiter Dynamic/2
  Unary Minus/1 -> Rate Limiter Dynamic/3
  Switch1/1 -> Unary Minus/1, Rate Limiter Dynamic/1
  huge/1 -> Switch1/1
  reset_high_active/1 -> Switch/2, Switch1/2
  initial_value/1 -> Switch/1
  rate/1 -> Switch1/3
  Rate Limiter Dynamic/1 -> y/1
  u/1 -> Switch/3

== system LOPES_3D/NMC Limiters - Click box/SmartRateLimit3/RateLimiterWithReset ==
  u : Inport
  rate : Inport  Port=2
  initial_value : Inport  Port=3
  reset_high_active : Inport  Port=4
  Rate Limiter Dynamic : simulink/Discontinuities/Rate Limiter Dynamic
  Switch : Switch  Criteria=u2 ~= 0
  Switch1 : Switch  Criteria=u2 ~= 0
  Unary Minus : UnaryMinus
  huge : Constant  Value=1e300
  y : Outport
  wires:
  u/1 -> Switch/3
  Rate Limiter Dynamic/1 -> y/1
  rate/1 -> Switch1/3
  initial_value/1 -> Switch/1
  reset_high_active/1 -> Switch1/2, Switch/2
  huge/1 -> Switch1/1
  Switch1/1 -> Rate Limiter Dynamic/1, Unary Minus/1
  Unary Minus/1 -> Rate Limiter Dynamic/3
  Switch/1 -> Rate Limiter Dynamic/2

== system LOPES_3D/NMC Limiters - Click box/SmartRateLimit4/RateLimiterWithReset ==
  u : Inport
  rate : Inport  Port=2
  initial_value : Inport  Port=3
  reset_high_active : Inport  Port=4
  Rate Limiter Dynamic : simulink/Discontinuities/Rate Limiter Dynamic
  Switch : Switch  Criteria=u2 ~= 0
  Switch1 : Switch  Criteria=u2 ~= 0
  Unary Minus : UnaryMinus
  huge : Constant  Value=1e300
  y : Outport
  wires:
  u/1 -> Switch/3
  Rate Limiter Dynamic/1 -> y/1
  rate/1 -> Switch1/3
  initial_value/1 -> Switch/1
  reset_high_active/1 -> Switch1/2, Switch/2
  huge/1 -> Switch1/1
  Switch1/1 -> Rate Limiter Dynamic/1, Unary Minus/1
  Unary Minus/1 -> Rate Limiter Dynamic/3
  Switch/1 -> Rate Limiter Dynamic/2

== system LOPES_3D/NMC Limiters - Click box/SmartRateLimit5/RateLimiterWithReset ==
  u : Inport
  rate : Inport  Port=2
  initial_value : Inport  Port=3
  reset_high_active : Inport  Port=4
  Rate Limiter Dynamic : simulink/Discontinuities/Rate Limiter Dynamic
  Switch : Switch  Criteria=u2 ~= 0
  Switch1 : Switch  Criteria=u2 ~= 0
  Unary Minus : UnaryMinus
  huge : Constant  Value=1e300
  y : Outport
  wires:
  Switch/1 -> Rate Limiter Dynamic/2
  Unary Minus/1 -> Rate Limiter Dynamic/3
  Switch1/1 -> Unary Minus/1, Rate Limiter Dynamic/1
  huge/1 -> Switch1/1
  reset_high_active/1 -> Switch/2, Switch1/2
  initial_value/1 -> Switch/1
  rate/1 -> Switch1/3
  Rate Limiter Dynamic/1 -> y/1
  u/1 -> Switch/3

== system LOPES_3D/NMC Limiters - Click box/SmartRateLimit6/RateLimiterWithReset ==
  u : Inport
  rate : Inport  Port=2
  initial_value : Inport  Port=3
  reset_high_active : Inport  Port=4
  Rate Limiter Dynamic : simulink/Discontinuities/Rate Limiter Dynamic
  Switch : Switch  Criteria=u2 ~= 0
  Switch1 : Switch  Criteria=u2 ~= 0
  Unary Minus : UnaryMinus
  huge : Constant  Value=1e300
  y : Outport
  wires:
  u/1 -> Switch/3
  Rate Limiter Dynamic/1 -> y/1
  rate/1 -> Switch1/3
  initial_value/1 -> Switch/1
  reset_high_active/1 -> Switch1/2, Switch/2
  huge/1 -> Switch1/1
  Switch1/1 -> Rate Limiter Dynamic/1, Unary Minus/1
  Unary Minus/1 -> Rate Limiter Dynamic/3
  Switch/1 -> Rate Limiter Dynamic/2

== stateflow chart LOPES_3D/StateDiagram ==
  state ActiveState
    state StartLeft
      entry:
      State = 201;
    state LonR
      entry:
      State = 101;
      DesState = InputState;
    state StoppingRight
      entry:
      State = 301;
    state StoppedRight
      entry:
      State = 401;
    state Init
    state SwingRight
      entry:
      State = 102;
    state SwingLeft
      entry:
      State = 104;
    state StartRight
      entry:
      State = 202;
    state RonL
      entry:
      State = 103;
      DesState = InputState;
    state StoppingLeft
      entry:
      State = 302;
    state StoppedLeft
      entry:
      State = 402;
    LonR -> StoppingRight [order 2] : [DesState == 3]
    SwingLeft -> LonR : [PhasePerc > 0 && PhasePerc < 2]
    StoppingRight -> StoppedRight : [PhasePerc > 50]
    StartLeft -> LonR : [PhasePerc > 0 && PhasePerc < 2]
    Init -> StartLeft [order 2] : [StartLeg == 1]
    LonR -> SwingRight [order 1] : [MeasPhase == 2&&DesState==2 ]
    (default) -> Init
    Init -> StartRight [order 1] : [StartLeg == 2]
    SwingRight -> RonL : [PhasePerc > 50]
    RonL -> SwingLeft [order 1] : [MeasPhase == 4 &&DesState==2 ]
    StoppingLeft -> StoppedLeft : [PhasePerc > 0 && PhasePerc < 2]
    StartRight -> RonL : [PhasePerc > 50&& PhasePerc < 52]
    RonL -> StoppingLeft [order 2] : [DesState == 3]
  state Start
    entry:
    if StartLeg == 1
    State = 501;
    elseif StartLeg == 2
    State = 502;
    end
    during:
    if StartLeg == 1
    State = 501;
    elseif StartLeg == 2
    State = 502;
    end
  StoppedRight -> Start : [InputState == 2]
  Start -> ActiveState : [InputState == 2]
  (default) -> Start
  ActiveState -> Start : [InputState == 1]
  StoppedLeft -> Start : [InputState == 2]
  data: InputState input; PhasePerc input; MeasPhase input; StartLeg input; State output; DesState local
